simulink model "Uebung07_Aufgabe1_nach_Fusion"  (R2016a)
settings: Solver=VariableStepAuto  StartTime=0.0  StopTime=10000  RelTol=1e-3
undefined symbols (not defined in the file or in its folder): calcElapsedTime, entity, m, n
settings Model: Creator=gome  LastModifiedBy=gome

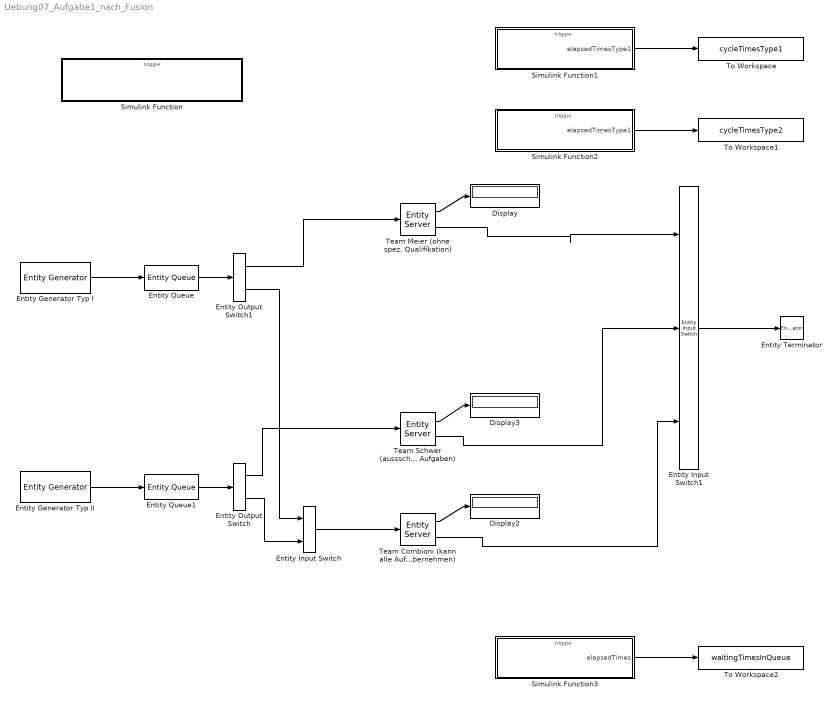
== system Uebung07_Aufgabe1_nach_Fusion ==
  Display : Display
  Display2 : Display
  Display3 : Display
  Entity Input Switch : EntityInputSwitch  InputPortMessageModes=m,m  OutputPortMessageModes=m
  Entity Input Switch1 : EntityInputSwitch  InputPortMessageModes=m,m,m  OutputPortMessageModes=m  NumberInputPorts=3
      settings: InputPortMap=u1,u2,u3
  Entity Output Switch : EntityOutputSwitch  InputPortMessageModes=m  OutputPortMessageModes=m,m  SwitchAttributeName=Attribute1
  Entity Output Switch1 : EntityOutputSwitch  InputPortMessageModes=m  OutputPortMessageModes=m,m  SwitchAttributeName=Attribute1
  Entity Generator Typ I : EntityGenerator  OutputPortMessageModes=m  TimeSource=MATLAB action  IntergenerationTimeAction=dt = exprnd(1/(49/12));  GenerateAction=|  AttributeName=startTime|serviceTime|type  AttributeInitialValue=1|1|1  EntityType=Structured  EntityTypeName=Entity
      | persistent init
      | if isempty(init)
      |     init = 1;
      |     rng(61351);
      | end
      | 
      | entity.startTime = getCurrentSimTime;
      | entity.serviceTime = exprnd(0.25);
  Entity Generator Typ II : EntityGenerator  OutputPortMessageModes=m  TimeSource=MATLAB action  Period=36.3636  IntergenerationTimeAction=|  GenerateAction=|  AttributeName=startTime|serviceTime|type  AttributeInitialValue=1|1|2  EntityType=Structured  EntityTypeName=Entity
      | persistent init
      | if isempty(init)
      |     init = 1;
      |     rng(4850);
      | end
      | 
      | dt = exprnd(1/(14/12));
      | persistent init
      | if isempty(init)
      |     init = 1;
      |     rng(35461654);
      | end
      | 
      | entity.startTime = getCurrentSimTime;
      | entity.serviceTime = exprnd(1);
  Entity Queue : EntityQueue  InputPortMessageModes=m  OutputPortMessageModes=m  Capacity=inf  ExitAction=calcElapsedTime(entity.startTime);
      settings: OutputPortMap=o5
  Entity Queue1 : EntityQueue  InputPortMessageModes=m  OutputPortMessageModes=m  Capacity=inf  ExitAction=calcElapsedTime(entity.startTime);
      settings: OutputPortMap=o5
  Entity Terminator : EntityTerminator  InputPortMessageModes=m  EntryAction=|
      | if entity.type == 1
      |     calcElapsedTime1(entity.startTime);
      | else
      |     calcElapsedTime2(entity.startTime);
      | end
  Simulink Function : Subsystem  TreatAsAtomicUnit=on
  Simulink Function1 : Subsystem  TreatAsAtomicUnit=on
  Simulink Function2 : Subsystem  TreatAsAtomicUnit=on
  Simulink Function3 : Subsystem  TreatAsAtomicUnit=on
  Team Combioni (kann alle Aufgaben übernehmen) : EntityServer  InputPortMessageModes=m  OutputPortMessageModes=n,m  Capacity=2  ServiceTimeSource=Attribute  ServiceTimeAttributeName=serviceTime  Utilization=on
      settings: OutputPortMap=o5,o9
  Team Meier (ohne spez. Qualifikation) : EntityServer  InputPortMessageModes=m  OutputPortMessageModes=n,m  Capacity=2  ServiceTimeSource=Attribute  ServiceTimeAttributeName=serviceTime  Utilization=on
      settings: OutputPortMap=o5,o9
  Team Schwer (aussschliesslich komplizerte Aufgaben) : EntityServer  InputPortMessageModes=m  OutputPortMessageModes=n,m  Capacity=1  ServiceTimeSource=Attribute  ServiceTimeAttributeName=serviceTime  Utilization=on
      settings: OutputPortMap=o5,o9
  To Workspace : ToWorkspace  VariableName=cycleTimesType1  SaveFormat=Timeseries  SampleTime=-1
  To Workspace1 : ToWorkspace  VariableName=cycleTimesType2  SaveFormat=Timeseries  SampleTime=-1
  To Workspace2 : ToWorkspace  VariableName=waitingTimesInQueue  SaveFormat=Timeseries  SampleTime=-1
  wires:
  Entity Queue/1 -> Entity Output Switch1/1
  Entity Queue1/1 -> Entity Output Switch/1
  Entity Generator Typ II/1 -> Entity Queue1/1
  Entity Generator Typ I/1 -> Entity Queue/1
  Entity Output Switch1/1 -> Team Meier (ohne spez. Qualifikation)/1
  Entity Output Switch1/2 -> Entity Input Switch/1
  Entity Output Switch/2 -> Entity Input Switch/2
  Team Meier (ohne spez. Qualifikation)/2 -> Entity Input Switch1/1
  Team Schwer (aussschliesslich komplizerte Aufgaben)/2 -> Entity Input Switch1/2
  Team Combioni (kann alle Aufgaben übernehmen)/2 -> Entity Input Switch1/3
  Entity Input Switch1/1 -> Entity Terminator/1
  Simulink Function1/1(elapsedTimesType1) -> To Workspace/1
  Team Meier (ohne spez. Qualifikation)/1 -> Display/1
  Team Combioni (kann alle Aufgaben übernehmen)/1 -> Display2/1
  Team Schwer (aussschliesslich komplizerte Aufgaben)/1 -> Display3/1
  Simulink Function2/1(elapsedTimesType1) -> To Workspace1/1
  Simulink Function3/1(elapsedTimes) -> To Workspace2/1
  Entity Input Switch/1 -> Team Combioni (kann alle Aufgaben übernehmen)/1
  Entity Output Switch/1 -> Team Schwer (aussschliesslich komplizerte Aufgaben)/1

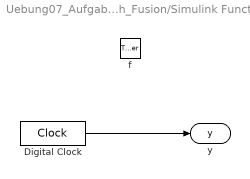
== system Uebung07_Aufgabe1_nach_Fusion/Simulink Function ==
  f : TriggerPort  TriggerType=function-call  IsSimulinkFunction=on  FunctionName=getCurrentSimTime  VariantControl=Variant
  Digital Clock : DigitalClock  SampleTime=-1
  y : ArgOut  DisableCoverage=on  ArgumentName=y
  wires:
  Digital Clock/1 -> y/1

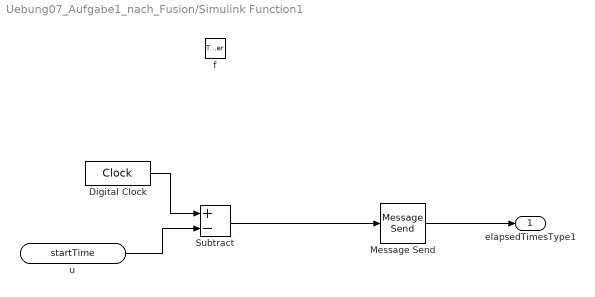
== system Uebung07_Aufgabe1_nach_Fusion/Simulink Function1 ==
  f : TriggerPort  TriggerType=function-call  IsSimulinkFunction=on  FunctionName=calcElapsedTime1  VariantControl=Variant
  Digital Clock : DigitalClock  SampleTime=-1
  Message Send : MessageSend  OutputPortMessageModes=m
      settings: InputPortMap=u1
  Subtract : Sum  Inputs=+-
  u : ArgIn  DisableCoverage=on  ArgumentName=startTime
  elapsedTimesType1 : Outport
  wires:
  Message Send/1 -> elapsedTimesType1/1
  Subtract/1 -> Message Send/1
  Digital Clock/1 -> Subtract/1
  u/1 -> Subtract/2

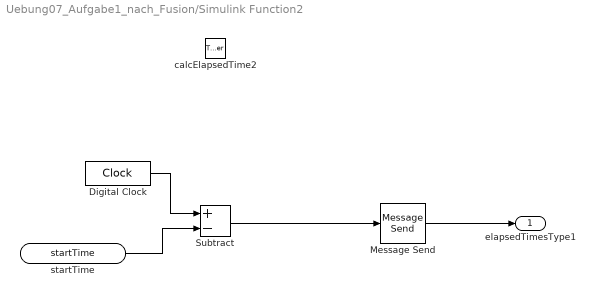
== system Uebung07_Aufgabe1_nach_Fusion/Simulink Function2 ==
  calcElapsedTime2 : TriggerPort  TriggerType=function-call  IsSimulinkFunction=on  FunctionName=calcElapsedTime2  VariantControl=Variant
  Digital Clock : DigitalClock  SampleTime=-1
  Message Send : MessageSend  OutputPortMessageModes=m
      settings: InputPortMap=u1
  Subtract : Sum  Inputs=+-
  startTime : ArgIn  DisableCoverage=on  ArgumentName=startTime
  elapsedTimesType1 : Outport
  wires:
  Message Send/1 -> elapsedTimesType1/1
  Subtract/1 -> Message Send/1
  Digital Clock/1 -> Subtract/1
  startTime/1 -> Subtract/2

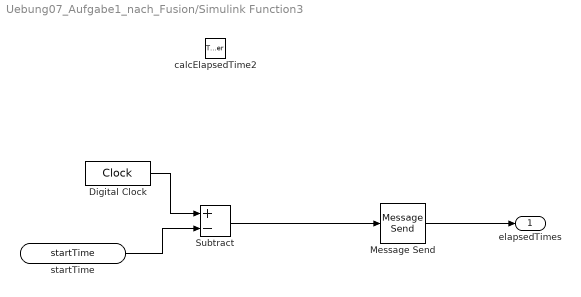
== system Uebung07_Aufgabe1_nach_Fusion/Simulink Function3 ==
  calcElapsedTime2 : TriggerPort  TriggerType=function-call  IsSimulinkFunction=on  FunctionName=calcElapsedTime  VariantControl=Variant
  Digital Clock : DigitalClock  SampleTime=-1
  Message Send : MessageSend  OutputPortMessageModes=m
      settings: InputPortMap=u1
  Subtract : Sum  Inputs=+-
  startTime : ArgIn  DisableCoverage=on  ArgumentName=startTime
  elapsedTimes : Outport
  wires:
  Message Send/1 -> elapsedTimes/1
  Subtract/1 -> Message Send/1
  Digital Clock/1 -> Subtract/1
  startTime/1 -> Subtract/2
